simulink model "LocalPlanner"  (R2023b)
settings: Solver=VariableStepAuto  StartTime=0.0  StopTime=tsReplan*2  RelTol=1e-3
undefined symbols (not defined in the file or in its folder): curpose, curvel, maxRefPathLen
settings Model: DataDictionary=PlannerData.sldd  Creator=cstabile  LastModifiedBy=cstabile
settings DataIOCC: SaveTime=off
settings SFSimCC: SimTargetLang=C++

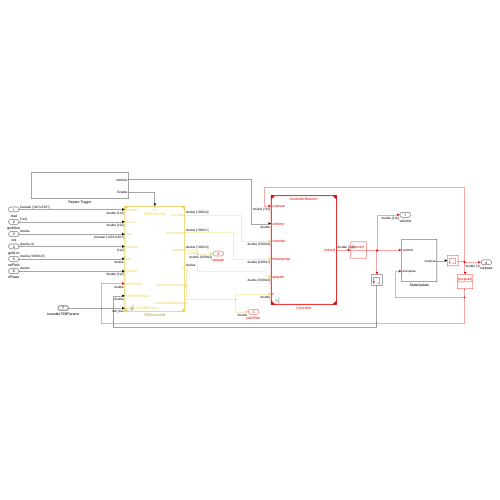
[thumbnail: Simulink's stored preview of the top-level diagram]
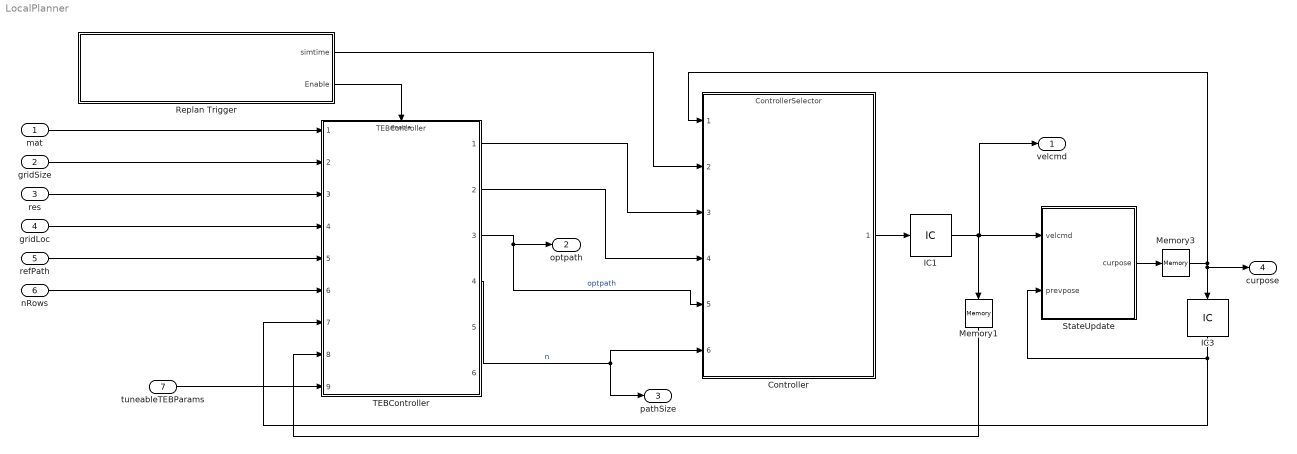
== system LocalPlanner ==
  mat : Inport  OutDataTypeStr=boolean  PortDimensions=[1201 1201]
  gridSize : Inport  Port=2  PortDimensions=[1 2]
  res : Inport  Port=3  OutDataTypeStr=double  PortDimensions=1
  gridLoc : Inport  Port=4  OutDataTypeStr=double  PortDimensions=2
  refPath : Inport  Port=5  OutDataTypeStr=double  PortDimensions=[maxRefPathLen 3]  Interpolate=off
  nRows : Inport  Port=6  OutDataTypeStr=double  PortDimensions=1  Interpolate=off
  tuneableTEBParams : Inport  Port=7  OutDataTypeStr=Bus: teb_bus  SampleTime=0  Interpolate=off
  Controller : ModelReference  ModelNameDialog=ControllerSelector  ModelReferenceVersion=2.0
  IC1 : InitialCondition  Value=curvel
  IC3 : InitialCondition  Value=curpose
  Memory1 : Memory  InheritSampleTime=on
  Memory3 : Memory  InheritSampleTime=on
  Replan Trigger : Subsystem  mask{replanInterval=3.0}
      mask prompts: replanInterval "Replan Interval (in seconds)"
  StateUpdate : Subsystem
  TEBController : ModelReference  ModelNameDialog=TEBController.slx  ModelReferenceVersion=2.2  EnablePortName=Enable  EnablePortStatesWhenEnabling=held
  velcmd : Outport  OutDataTypeStr=double  PortDimensions=[1 2]  SampleTime=[0.001,0]
  optpath : Outport  Port=2  OutDataTypeStr=double  PortDimensions=[1000 3]  SampleTime=[0.001,0]
  pathSize : Outport  Port=3  OutDataTypeStr=double  PortDimensions=1  SampleTime=[0.001,0]
  curpose : Outport  Port=4  OutDataTypeStr=double  PortDimensions=3  SampleTime=[0.001,0]
  wires:
  TEBController/3 -> Controller/5, optpath/1  "optpath"
  Memory1/1 -> TEBController/8
  refPath/1 -> TEBController/5
  Memory3/1 -> Controller/1, IC3/1, curpose/1
  TEBController/1 -> Controller/3
  nRows/1 -> TEBController/6
  TEBController/4 -> Controller/6, pathSize/1  "n"
  TEBController/2 -> Controller/4
  res/1 -> TEBController/3
  gridLoc/1 -> TEBController/4
  mat/1 -> TEBController/1
  Replan Trigger/2(Enable) -> TEBController/Enable
  Replan Trigger/1(simtime) -> Controller/2
  Controller/1 -> IC1/1
  StateUpdate/1(curpose) -> Memory3/1
  IC3/1 -> TEBController/7, StateUpdate/2(prevpose)
  IC1/1 -> StateUpdate/1(velcmd), velcmd/1, Memory1/1
  tuneableTEBParams/1 -> TEBController/9
  gridSize/1 -> TEBController/2

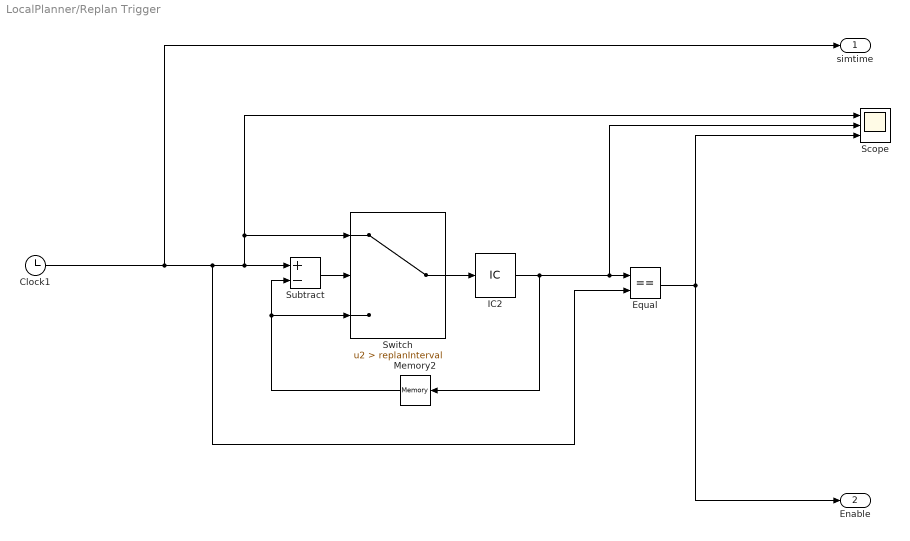
== system LocalPlanner/Replan Trigger ==
  Clock1 : Clock
  Equal : RelationalOperator  Operator===  OutDataTypeStr=boolean  RndMeth=Simplest  InputSameDT=off
  IC2 : InitialCondition  Value=0
  Memory2 : Memory
  Scope : Scope  NumInputPorts=3
  Subtract : Sum  Inputs=+-
  Switch : Switch  Criteria=u2 > Threshold  Threshold=replanInterval  SaturateOnIntegerOverflow=off  InputSameDT=off
  simtime : Outport
  Enable : Outport  Port=2
  wires:
  Clock1/1 -> simtime/1, Subtract/1, Switch/1, Scope/1, Equal/2
  IC2/1 -> Equal/1, Scope/2, Memory2/1
  Subtract/1 -> Switch/2
  Switch/1 -> IC2/1
  Memory2/1 -> Subtract/2, Switch/3
  Equal/1 -> Enable/1, Scope/3

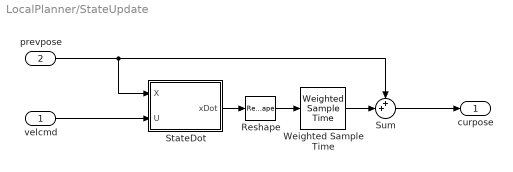
== system LocalPlanner/StateUpdate ==
  velcmd : Inport
  prevpose : Inport  Port=2
  Reshape : Reshape  OutputDimensionality=Row vector (2-D)
  StateDot : MATLAB Function  TreatAsAtomicUnit=on
  Sum : Sum  Inputs=++|
  Weighted Sample Time : WeightedSampleTime  TsampMathOp=*
  curpose : Outport
  wires:
  Weighted Sample Time/1 -> Sum/2
  StateDot/1(xDot) -> Reshape/1
  velcmd/1 -> StateDot/2(U)
  prevpose/1 -> Sum/1, StateDot/1(X)
  Sum/1 -> curpose/1
  Reshape/1 -> Weighted Sample Time/1

== matlab function LocalPlanner/StateUpdate/StateDot ==
  settings: updateMethod=DISCRETE  sampleTime=tsIntegrator
  data: X input; xDot output; U input
function xDot = xdot(X,U)
    % X = [x y theta]
    % U = [vel angVel]
    xDot = [
        cos(X(3))*U(1)     % dx/dt
        sin(X(3))*U(1)     % dy/dt 
        U(2)];              % dtheta/dt
end
